simulink model "aa_IOT"  (R2024b)
settings: Solver=VariableStepAuto  StartTime=0.0  StopTime=0.20  RelTol=1e-3
undefined symbols (not defined in the file): Acid, Ion, Lead, Lithium, sigbuilder_block
libraries: spsBreakerLib x120, spsBatteryLib x72, spsSeriesRLCBranchLib x47, spsVoltageMeasurementLib x33, spsIdealSwitchLib x19, spsDiodeLib x10, spsCurrentMeasurementLib x8, spsThyristorLib x6, sldrtlib x4, spsACVoltageSourceLib x3, spsIGBTLib x2, spsPVArrayLib x1
(part 6 of 7)

== matlab function aa_IOT/Subsystem11/Swapping battery controller/MATLAB Function12 ==
  settings: updateMethod=DISCRETE
  data: SOC input; LoadOn output; ChargingOn output
function [LoadOn, ChargingOn] = chargeDischargeNode(SOC)
    % This function determines the charging and discharging states
    % based on the state of charge (SOC) of the battery.
    % Inputs:
    %   SOC - Current state of charge (0 to 100)
    % Outputs:
    %   LoadOn - Indicator if the load is on (1) or off (0)
    %   ChargingOn - Indicator if charging is active (1) or not (0)

    % Initialize persistent variables to retain state across function calls
    persistent LoadOnPersistent;
    persistent ChargingOnPersistent;

    if isempty(LoadOnPersistent)  % Initialize on first call
        LoadOnPersistent = 1;     % Load is initially on
        ChargingOnPersistent = 0;  % Charging is initially off
    end

    % Logic for charging and discharging based on SOC levels
    if SOC > 80
        LoadOnPersistent = 1;      % Turn load on if SOC is above 80%
        ChargingOnPersistent = 0;   % Turn charging off
    elseif SOC < 40
        LoadOnPersistent = 0;      % Turn load off if SOC is below 40%
        ChargingOnPersistent = 1;   % Start charging
    end

    % Assign output values from persistent variables
    LoadOn = LoadOnPersistent;
    ChargingOn = ChargingOnPersistent;
end

== matlab function aa_IOT/Subsystem11/Swapping battery controller/MATLAB Function13 ==
  settings: updateMethod=DISCRETE
  data: SOC input; LoadOn output; ChargingOn output
function [LoadOn, ChargingOn] = chargeDischargeNode(SOC)
    % This function determines the charging and discharging states
    % based on the state of charge (SOC) of the battery.
    % Inputs:
    %   SOC - Current state of charge (0 to 100)
    % Outputs:
    %   LoadOn - Indicator if the load is on (1) or off (0)
    %   ChargingOn - Indicator if charging is active (1) or not (0)

    % Initialize persistent variables to retain state across function calls
    persistent LoadOnPersistent;
    persistent ChargingOnPersistent;

    if isempty(LoadOnPersistent)  % Initialize on first call
        LoadOnPersistent = 1;     % Load is initially on
        ChargingOnPersistent = 0;  % Charging is initially off
    end

    % Logic for charging and discharging based on SOC levels
    if SOC > 80
        LoadOnPersistent = 1;      % Turn load on if SOC is above 80%
        ChargingOnPersistent = 0;   % Turn charging off
    elseif SOC < 40
        LoadOnPersistent = 0;      % Turn load off if SOC is below 40%
        ChargingOnPersistent = 1;   % Start charging
    end

    % Assign output values from persistent variables
    LoadOn = LoadOnPersistent;
    ChargingOn = ChargingOnPersistent;
end

== matlab function aa_IOT/Subsystem11/Swapping battery controller/MATLAB Function14 ==
  settings: updateMethod=DISCRETE
  data: SOC input; LoadOn output; ChargingOn output
function [LoadOn, ChargingOn] = chargeDischargeNode(SOC)
    % This function determines the charging and discharging states
    % based on the state of charge (SOC) of the battery.
    % Inputs:
    %   SOC - Current state of charge (0 to 100)
    % Outputs:
    %   LoadOn - Indicator if the load is on (1) or off (0)
    %   ChargingOn - Indicator if charging is active (1) or not (0)

    % Initialize persistent variables to retain state across function calls
    persistent LoadOnPersistent;
    persistent ChargingOnPersistent;

    if isempty(LoadOnPersistent)  % Initialize on first call
        LoadOnPersistent = 1;     % Load is initially on
        ChargingOnPersistent = 0;  % Charging is initially off
    end

    % Logic for charging and discharging based on SOC levels
    if SOC > 80
        LoadOnPersistent = 1;      % Turn load on if SOC is above 80%
        ChargingOnPersistent = 0;   % Turn charging off
    elseif SOC < 40
        LoadOnPersistent = 0;      % Turn load off if SOC is below 40%
        ChargingOnPersistent = 1;   % Start charging
    end

    % Assign output values from persistent variables
    LoadOn = LoadOnPersistent;
    ChargingOn = ChargingOnPersistent;
end

== matlab function aa_IOT/Subsystem11/Swapping battery controller/MATLAB Function15 ==
  settings: updateMethod=DISCRETE
  data: SOC input; LoadOn output; ChargingOn output
function [LoadOn, ChargingOn] = chargeDischargeNode(SOC)
    % This function determines the charging and discharging states
    % based on the state of charge (SOC) of the battery.
    % Inputs:
    %   SOC - Current state of charge (0 to 100)
    % Outputs:
    %   LoadOn - Indicator if the load is on (1) or off (0)
    %   ChargingOn - Indicator if charging is active (1) or not (0)

    % Initialize persistent variables to retain state across function calls
    persistent LoadOnPersistent;
    persistent ChargingOnPersistent;

    if isempty(LoadOnPersistent)  % Initialize on first call
        LoadOnPersistent = 1;     % Load is initially on
        ChargingOnPersistent = 0;  % Charging is initially off
    end

    % Logic for charging and discharging based on SOC levels
    if SOC > 80
        LoadOnPersistent = 1;      % Turn load on if SOC is above 80%
        ChargingOnPersistent = 0;   % Turn charging off
    elseif SOC < 40
        LoadOnPersistent = 0;      % Turn load off if SOC is below 40%
        ChargingOnPersistent = 1;   % Start charging
    end

    % Assign output values from persistent variables
    LoadOn = LoadOnPersistent;
    ChargingOn = ChargingOnPersistent;
end

== matlab function aa_IOT/Subsystem11/Swapping battery controller/MATLAB Function16 ==
  settings: updateMethod=DISCRETE
  data: SOC input; LoadOn output; ChargingOn output
function [LoadOn, ChargingOn] = chargeDischargeNode(SOC)
    % This function determines the charging and discharging states
    % based on the state of charge (SOC) of the battery.
    % Inputs:
    %   SOC - Current state of charge (0 to 100)
    % Outputs:
    %   LoadOn - Indicator if the load is on (1) or off (0)
    %   ChargingOn - Indicator if charging is active (1) or not (0)

    % Initialize persistent variables to retain state across function calls
    persistent LoadOnPersistent;
    persistent ChargingOnPersistent;

    if isempty(LoadOnPersistent)  % Initialize on first call
        LoadOnPersistent = 1;     % Load is initially on
        ChargingOnPersistent = 0;  % Charging is initially off
    end

    % Logic for charging and discharging based on SOC levels
    if SOC > 80
        LoadOnPersistent = 1;      % Turn load on if SOC is above 80%
        ChargingOnPersistent = 0;   % Turn charging off
    elseif SOC < 40
        LoadOnPersistent = 0;      % Turn load off if SOC is below 40%
        ChargingOnPersistent = 1;   % Start charging
    end

    % Assign output values from persistent variables
    LoadOn = LoadOnPersistent;
    ChargingOn = ChargingOnPersistent;
end

== matlab function aa_IOT/Subsystem11/Swapping battery controller/MATLAB Function17 ==
  settings: updateMethod=DISCRETE
  data: SOC input; LoadOn output; ChargingOn output
function [LoadOn, ChargingOn] = chargeDischargeNode(SOC)
    % This function determines the charging and discharging states
    % based on the state of charge (SOC) of the battery.
    % Inputs:
    %   SOC - Current state of charge (0 to 100)
    % Outputs:
    %   LoadOn - Indicator if the load is on (1) or off (0)
    %   ChargingOn - Indicator if charging is active (1) or not (0)

    % Initialize persistent variables to retain state across function calls
    persistent LoadOnPersistent;
    persistent ChargingOnPersistent;

    if isempty(LoadOnPersistent)  % Initialize on first call
        LoadOnPersistent = 1;     % Load is initially on
        ChargingOnPersistent = 0;  % Charging is initially off
    end

    % Logic for charging and discharging based on SOC levels
    if SOC > 80
        LoadOnPersistent = 1;      % Turn load on if SOC is above 80%
        ChargingOnPersistent = 0;   % Turn charging off
    elseif SOC < 40
        LoadOnPersistent = 0;      % Turn load off if SOC is below 40%
        ChargingOnPersistent = 1;   % Start charging
    end

    % Assign output values from persistent variables
    LoadOn = LoadOnPersistent;
    ChargingOn = ChargingOnPersistent;
end

== matlab function aa_IOT/Subsystem11/Swapping battery controller/MATLAB Function18 ==
  settings: updateMethod=DISCRETE
  data: SOC input; LoadOn output; ChargingOn output
function [LoadOn, ChargingOn] = chargeDischargeNode(SOC)
    % This function determines the charging and discharging states
    % based on the state of charge (SOC) of the battery.
    % Inputs:
    %   SOC - Current state of charge (0 to 100)
    % Outputs:
    %   LoadOn - Indicator if the load is on (1) or off (0)
    %   ChargingOn - Indicator if charging is active (1) or not (0)

    % Initialize persistent variables to retain state across function calls
    persistent LoadOnPersistent;
    persistent ChargingOnPersistent;

    if isempty(LoadOnPersistent)  % Initialize on first call
        LoadOnPersistent = 1;     % Load is initially on
        ChargingOnPersistent = 0;  % Charging is initially off
    end

    % Logic for charging and discharging based on SOC levels
    if SOC > 80
        LoadOnPersistent = 1;      % Turn load on if SOC is above 80%
        ChargingOnPersistent = 0;   % Turn charging off
    elseif SOC < 40
        LoadOnPersistent = 0;      % Turn load off if SOC is below 40%
        ChargingOnPersistent = 1;   % Start charging
    end

    % Assign output values from persistent variables
    LoadOn = LoadOnPersistent;
    ChargingOn = ChargingOnPersistent;
end

== matlab function aa_IOT/Subsystem11/Swapping battery controller/MATLAB Function19 ==
  settings: updateMethod=DISCRETE
  data: SOC input; LoadOn output; ChargingOn output
function [LoadOn, ChargingOn] = chargeDischargeNode(SOC)
    % This function determines the charging and discharging states
    % based on the state of charge (SOC) of the battery.
    % Inputs:
    %   SOC - Current state of charge (0 to 100)
    % Outputs:
    %   LoadOn - Indicator if the load is on (1) or off (0)
    %   ChargingOn - Indicator if charging is active (1) or not (0)

    % Initialize persistent variables to retain state across function calls
    persistent LoadOnPersistent;
    persistent ChargingOnPersistent;

    if isempty(LoadOnPersistent)  % Initialize on first call
        LoadOnPersistent = 1;     % Load is initially on
        ChargingOnPersistent = 0;  % Charging is initially off
    end

    % Logic for charging and discharging based on SOC levels
    if SOC > 80
        LoadOnPersistent = 1;      % Turn load on if SOC is above 80%
        ChargingOnPersistent = 0;   % Turn charging off
    elseif SOC < 40
        LoadOnPersistent = 0;      % Turn load off if SOC is below 40%
        ChargingOnPersistent = 1;   % Start charging
    end

    % Assign output values from persistent variables
    LoadOn = LoadOnPersistent;
    ChargingOn = ChargingOnPersistent;
end

== matlab function aa_IOT/Subsystem11/Swapping battery controller/MATLAB Function20 ==
  settings: updateMethod=DISCRETE
  data: SOC input; LoadOn output; ChargingOn output
function [LoadOn, ChargingOn] = chargeDischargeNode(SOC)
    % This function determines the charging and discharging states
    % based on the state of charge (SOC) of the battery.
    % Inputs:
    %   SOC - Current state of charge (0 to 100)
    % Outputs:
    %   LoadOn - Indicator if the load is on (1) or off (0)
    %   ChargingOn - Indicator if charging is active (1) or not (0)

    % Initialize persistent variables to retain state across function calls
    persistent LoadOnPersistent;
    persistent ChargingOnPersistent;

    if isempty(LoadOnPersistent)  % Initialize on first call
        LoadOnPersistent = 1;     % Load is initially on
        ChargingOnPersistent = 0;  % Charging is initially off
    end

    % Logic for charging and discharging based on SOC levels
    if SOC > 80
        LoadOnPersistent = 1;      % Turn load on if SOC is above 80%
        ChargingOnPersistent = 0;   % Turn charging off
    elseif SOC < 40
        LoadOnPersistent = 0;      % Turn load off if SOC is below 40%
        ChargingOnPersistent = 1;   % Start charging
    end

    % Assign output values from persistent variables
    LoadOn = LoadOnPersistent;
    ChargingOn = ChargingOnPersistent;
end

== matlab function aa_IOT/Subsystem11/Swapping battery controller/MATLAB Function21 ==
  settings: updateMethod=DISCRETE
  data: SOC input; LoadOn output; ChargingOn output
function [LoadOn, ChargingOn] = chargeDischargeNode(SOC)
    % This function determines the charging and discharging states
    % based on the state of charge (SOC) of the battery.
    % Inputs:
    %   SOC - Current state of charge (0 to 100)
    % Outputs:
    %   LoadOn - Indicator if the load is on (1) or off (0)
    %   ChargingOn - Indicator if charging is active (1) or not (0)

    % Initialize persistent variables to retain state across function calls
    persistent LoadOnPersistent;
    persistent ChargingOnPersistent;

    if isempty(LoadOnPersistent)  % Initialize on first call
        LoadOnPersistent = 1;     % Load is initially on
        ChargingOnPersistent = 0;  % Charging is initially off
    end

    % Logic for charging and discharging based on SOC levels
    if SOC > 80
        LoadOnPersistent = 1;      % Turn load on if SOC is above 80%
        ChargingOnPersistent = 0;   % Turn charging off
    elseif SOC < 40
        LoadOnPersistent = 0;      % Turn load off if SOC is below 40%
        ChargingOnPersistent = 1;   % Start charging
    end

    % Assign output values from persistent variables
    LoadOn = LoadOnPersistent;
    ChargingOn = ChargingOnPersistent;
end

== matlab function aa_IOT/Subsystem11/Swapping battery controller/MATLAB Function22 ==
  settings: updateMethod=DISCRETE
  data: SOC input; LoadOn output; ChargingOn output
function [LoadOn, ChargingOn] = chargeDischargeNode(SOC)
    % This function determines the charging and discharging states
    % based on the state of charge (SOC) of the battery.
    % Inputs:
    %   SOC - Current state of charge (0 to 100)
    % Outputs:
    %   LoadOn - Indicator if the load is on (1) or off (0)
    %   ChargingOn - Indicator if charging is active (1) or not (0)

    % Initialize persistent variables to retain state across function calls
    persistent LoadOnPersistent;
    persistent ChargingOnPersistent;

    if isempty(LoadOnPersistent)  % Initialize on first call
        LoadOnPersistent = 1;     % Load is initially on
        ChargingOnPersistent = 0;  % Charging is initially off
    end

    % Logic for charging and discharging based on SOC levels
    if SOC > 80
        LoadOnPersistent = 1;      % Turn load on if SOC is above 80%
        ChargingOnPersistent = 0;   % Turn charging off
    elseif SOC < 40
        LoadOnPersistent = 0;      % Turn load off if SOC is below 40%
        ChargingOnPersistent = 1;   % Start charging
    end

    % Assign output values from persistent variables
    LoadOn = LoadOnPersistent;
    ChargingOn = ChargingOnPersistent;
end

== matlab function aa_IOT/Subsystem11/Subsystem5/MATLAB Function ==
  data: SOC input; output output; Voltage input; Current input
function output = checkBatteryStatus(SOC, Voltage, Current)
    % Check if the inputs are valid
    if SOC <= 0 || Voltage <= 0 || Current <= 0
        output = 0; % Return 0 if any input is less than or equal to 0
        return;
    end
    
    % Define threshold values
    SOC_threshold = 80; % in percentage
    Voltage_threshold = 10; % in volts
    Current_threshold = 13; % in amperes

    % Check conditions and return output
    if SOC > SOC_threshold && Voltage > Voltage_threshold && Current > Current_threshold
        output = 0; % Return 0 if all conditions are met
    else
        output = 1; % Return 1 otherwise
    end
end

== matlab function aa_IOT/Subsystem11/Swapping battery controller/MATLAB Function23 ==
  settings: updateMethod=DISCRETE
  data: SOC input; LoadOn output; ChargingOn output
function [LoadOn, ChargingOn] = chargeDischargeNode(SOC)
    % This function determines the charging and discharging states
    % based on the state of charge (SOC) of the battery.
    % Inputs:
    %   SOC - Current state of charge (0 to 100)
    % Outputs:
    %   LoadOn - Indicator if the load is on (1) or off (0)
    %   ChargingOn - Indicator if charging is active (1) or not (0)

    % Initialize persistent variables to retain state across function calls
    persistent LoadOnPersistent;
    persistent ChargingOnPersistent;

    if isempty(LoadOnPersistent)  % Initialize on first call
        LoadOnPersistent = 1;     % Load is initially on
        ChargingOnPersistent = 0;  % Charging is initially off
    end

    % Logic for charging and discharging based on SOC levels
    if SOC > 80
        LoadOnPersistent = 1;      % Turn load on if SOC is above 80%
        ChargingOnPersistent = 0;   % Turn charging off
    elseif SOC < 40
        LoadOnPersistent = 0;      % Turn load off if SOC is below 40%
        ChargingOnPersistent = 1;   % Start charging
    end

    % Assign output values from persistent variables
    LoadOn = LoadOnPersistent;
    ChargingOn = ChargingOnPersistent;
end

== matlab function aa_IOT/Subsystem11/Swapping battery controller/MATLAB Function24 ==
  settings: updateMethod=DISCRETE
  data: SOC input; LoadOn output; ChargingOn output
function [LoadOn, ChargingOn] = chargeDischargeNode(SOC)
    % This function determines the charging and discharging states
    % based on the state of charge (SOC) of the battery.
    % Inputs:
    %   SOC - Current state of charge (0 to 100)
    % Outputs:
    %   LoadOn - Indicator if the load is on (1) or off (0)
    %   ChargingOn - Indicator if charging is active (1) or not (0)

    % Initialize persistent variables to retain state across function calls
    persistent LoadOnPersistent;
    persistent ChargingOnPersistent;

    if isempty(LoadOnPersistent)  % Initialize on first call
        LoadOnPersistent = 1;     % Load is initially on
        ChargingOnPersistent = 0;  % Charging is initially off
    end

    % Logic for charging and discharging based on SOC levels
    if SOC > 80
        LoadOnPersistent = 1;      % Turn load on if SOC is above 80%
        ChargingOnPersistent = 0;   % Turn charging off
    elseif SOC < 40
        LoadOnPersistent = 0;      % Turn load off if SOC is below 40%
        ChargingOnPersistent = 1;   % Start charging
    end

    % Assign output values from persistent variables
    LoadOn = LoadOnPersistent;
    ChargingOn = ChargingOnPersistent;
end

== matlab function aa_IOT/Subsystem11/Swapping battery controller/MATLAB Function25 ==
  settings: updateMethod=DISCRETE
  data: SOC input; LoadOn output; ChargingOn output
function [LoadOn, ChargingOn] = chargeDischargeNode(SOC)
    % This function determines the charging and discharging states
    % based on the state of charge (SOC) of the battery.
    % Inputs:
    %   SOC - Current state of charge (0 to 100)
    % Outputs:
    %   LoadOn - Indicator if the load is on (1) or off (0)
    %   ChargingOn - Indicator if charging is active (1) or not (0)

    % Initialize persistent variables to retain state across function calls
    persistent LoadOnPersistent;
    persistent ChargingOnPersistent;

    if isempty(LoadOnPersistent)  % Initialize on first call
        LoadOnPersistent = 1;     % Load is initially on
        ChargingOnPersistent = 0;  % Charging is initially off
    end

    % Logic for charging and discharging based on SOC levels
    if SOC > 80
        LoadOnPersistent = 1;      % Turn load on if SOC is above 80%
        ChargingOnPersistent = 0;   % Turn charging off
    elseif SOC < 40
        LoadOnPersistent = 0;      % Turn load off if SOC is below 40%
        ChargingOnPersistent = 1;   % Start charging
    end

    % Assign output values from persistent variables
    LoadOn = LoadOnPersistent;
    ChargingOn = ChargingOnPersistent;
end

== matlab function aa_IOT/Subsystem11/Swapping battery controller/MATLAB Function26 ==
  settings: updateMethod=DISCRETE
  data: SOC input; LoadOn output; ChargingOn output
function [LoadOn, ChargingOn] = chargeDischargeNode(SOC)
    % This function determines the charging and discharging states
    % based on the state of charge (SOC) of the battery.
    % Inputs:
    %   SOC - Current state of charge (0 to 100)
    % Outputs:
    %   LoadOn - Indicator if the load is on (1) or off (0)
    %   ChargingOn - Indicator if charging is active (1) or not (0)

    % Initialize persistent variables to retain state across function calls
    persistent LoadOnPersistent;
    persistent ChargingOnPersistent;

    if isempty(LoadOnPersistent)  % Initialize on first call
        LoadOnPersistent = 1;     % Load is initially on
        ChargingOnPersistent = 0;  % Charging is initially off
    end

    % Logic for charging and discharging based on SOC levels
    if SOC > 80
        LoadOnPersistent = 1;      % Turn load on if SOC is above 80%
        ChargingOnPersistent = 0;   % Turn charging off
    elseif SOC < 40
        LoadOnPersistent = 0;      % Turn load off if SOC is below 40%
        ChargingOnPersistent = 1;   % Start charging
    end

    % Assign output values from persistent variables
    LoadOn = LoadOnPersistent;
    ChargingOn = ChargingOnPersistent;
end

== matlab function aa_IOT/Subsystem11/Swapping battery controller/MATLAB Function27 ==
  settings: updateMethod=DISCRETE
  data: SOC input; LoadOn output; ChargingOn output
function [LoadOn, ChargingOn] = chargeDischargeNode(SOC)
    % This function determines the charging and discharging states
    % based on the state of charge (SOC) of the battery.
    % Inputs:
    %   SOC - Current state of charge (0 to 100)
    % Outputs:
    %   LoadOn - Indicator if the load is on (1) or off (0)
    %   ChargingOn - Indicator if charging is active (1) or not (0)

    % Initialize persistent variables to retain state across function calls
    persistent LoadOnPersistent;
    persistent ChargingOnPersistent;

    if isempty(LoadOnPersistent)  % Initialize on first call
        LoadOnPersistent = 1;     % Load is initially on
        ChargingOnPersistent = 0;  % Charging is initially off
    end

    % Logic for charging and discharging based on SOC levels
    if SOC > 80
        LoadOnPersistent = 1;      % Turn load on if SOC is above 80%
        ChargingOnPersistent = 0;   % Turn charging off
    elseif SOC < 40
        LoadOnPersistent = 0;      % Turn load off if SOC is below 40%
        ChargingOnPersistent = 1;   % Start charging
    end

    % Assign output values from persistent variables
    LoadOn = LoadOnPersistent;
    ChargingOn = ChargingOnPersistent;
end

== matlab function aa_IOT/Subsystem11/Swapping battery controller/MATLAB Function28 ==
  settings: updateMethod=DISCRETE
  data: SOC input; LoadOn output; ChargingOn output
function [LoadOn, ChargingOn] = chargeDischargeNode(SOC)
    % This function determines the charging and discharging states
    % based on the state of charge (SOC) of the battery.
    % Inputs:
    %   SOC - Current state of charge (0 to 100)
    % Outputs:
    %   LoadOn - Indicator if the load is on (1) or off (0)
    %   ChargingOn - Indicator if charging is active (1) or not (0)

    % Initialize persistent variables to retain state across function calls
    persistent LoadOnPersistent;
    persistent ChargingOnPersistent;

    if isempty(LoadOnPersistent)  % Initialize on first call
        LoadOnPersistent = 1;     % Load is initially on
        ChargingOnPersistent = 0;  % Charging is initially off
    end

    % Logic for charging and discharging based on SOC levels
    if SOC > 80
        LoadOnPersistent = 1;      % Turn load on if SOC is above 80%
        ChargingOnPersistent = 0;   % Turn charging off
    elseif SOC < 40
        LoadOnPersistent = 0;      % Turn load off if SOC is below 40%
        ChargingOnPersistent = 1;   % Start charging
    end

    % Assign output values from persistent variables
    LoadOn = LoadOnPersistent;
    ChargingOn = ChargingOnPersistent;
end

== matlab function aa_IOT/Subsystem11/Swapping battery controller/MATLAB Function29 ==
  settings: updateMethod=DISCRETE
  data: SOC input; LoadOn output; ChargingOn output
function [LoadOn, ChargingOn] = chargeDischargeNode(SOC)
    % This function determines the charging and discharging states
    % based on the state of charge (SOC) of the battery.
    % Inputs:
    %   SOC - Current state of charge (0 to 100)
    % Outputs:
    %   LoadOn - Indicator if the load is on (1) or off (0)
    %   ChargingOn - Indicator if charging is active (1) or not (0)

    % Initialize persistent variables to retain state across function calls
    persistent LoadOnPersistent;
    persistent ChargingOnPersistent;

    if isempty(LoadOnPersistent)  % Initialize on first call
        LoadOnPersistent = 1;     % Load is initially on
        ChargingOnPersistent = 0;  % Charging is initially off
    end

    % Logic for charging and discharging based on SOC levels
    if SOC > 80
        LoadOnPersistent = 1;      % Turn load on if SOC is above 80%
        ChargingOnPersistent = 0;   % Turn charging off
    elseif SOC < 40
        LoadOnPersistent = 0;      % Turn load off if SOC is below 40%
        ChargingOnPersistent = 1;   % Start charging
    end

    % Assign output values from persistent variables
    LoadOn = LoadOnPersistent;
    ChargingOn = ChargingOnPersistent;
end

== matlab function aa_IOT/Subsystem11/Subsystem3/MATLAB Function ==
  data: SOC input; output output; Voltage input; Current input
function output = checkBatteryStatus(SOC, Voltage, Current)
    % Check if the inputs are valid
    if SOC <= 0 || Voltage <= 0 || Current <= 0
        output = 0; % Return 0 if any input is less than or equal to 0
        return;
    end
    
    % Define threshold values
    SOC_threshold = 80; % in percentage
    Voltage_threshold = 10; % in volts
    Current_threshold = 13; % in amperes

    % Check conditions and return output
    if SOC > SOC_threshold && Voltage > Voltage_threshold && Current > Current_threshold
        output = 0; % Return 0 if all conditions are met
    else
        output = 1; % Return 1 otherwise
    end
end

== matlab function aa_IOT/Subsystem11/Subsystem2/MATLAB Function ==
  data: SOC input; output output; Voltage input; Current input
function output = checkBatteryStatus(SOC, Voltage, Current)
    % Check if the inputs are valid
    if SOC <= 0 || Voltage <= 0 || Current <= 0
        output = 0; % Return 0 if any input is less than or equal to 0
        return;
    end
    
    % Define threshold values
    SOC_threshold = 80; % in percentage
    Voltage_threshold = 10; % in volts
    Current_threshold = 13; % in amperes

    % Check conditions and return output
    if SOC > SOC_threshold && Voltage > Voltage_threshold && Current > Current_threshold
        output = 0; % Return 0 if all conditions are met
    else
        output = 1; % Return 1 otherwise
    end
end

== matlab function aa_IOT/Subsystem11/Subsystem20/MATLAB Function ==
  data: SOC input; output output; Voltage input; Current input
function output = checkBatteryStatus(SOC, Voltage, Current)
    % Check if the inputs are valid
    if SOC <= 0 || Voltage <= 0 || Current <= 0
        output = 0; % Return 0 if any input is less than or equal to 0
        return;
    end
    
    % Define threshold values
    SOC_threshold = 80; % in percentage
    Voltage_threshold = 10; % in volts
    Current_threshold = 13; % in amperes

    % Check conditions and return output
    if SOC > SOC_threshold && Voltage > Voltage_threshold && Current > Current_threshold
        output = 0; % Return 0 if all conditions are met
    else
        output = 1; % Return 1 otherwise
    end
end

== matlab function aa_IOT/Subsystem11/Subsystem19/MATLAB Function ==
  data: SOC input; output output; Voltage input; Current input
function output = checkBatteryStatus(SOC, Voltage, Current)
    % Check if the inputs are valid
    if SOC <= 0 || Voltage <= 0 || Current <= 0
        output = 0; % Return 0 if any input is less than or equal to 0
        return;
    end
    
    % Define threshold values
    SOC_threshold = 80; % in percentage
    Voltage_threshold = 10; % in volts
    Current_threshold = 13; % in amperes

    % Check conditions and return output
    if SOC > SOC_threshold && Voltage > Voltage_threshold && Current > Current_threshold
        output = 0; % Return 0 if all conditions are met
    else
        output = 1; % Return 1 otherwise
    end
end

== matlab function aa_IOT/Solar/MPPT/Embedded MATLAB Function1 ==
  settings: updateMethod=DISCRETE
  data: V input; I input; T input; D output
function D   = PO(V,I,T)
persistent P2  P1  dP d dd n;
if isempty(V)
    V=370;
end
if isempty(I)
    I=0;
end
if isempty(P2)
    P2=0;
end
if isempty(P1)
    P1=0;
end
if isempty(dP)
    dP=0;
end
if isempty(d)
    d=1;
end
if isempty(dd)
    dd=0;
end
if isempty(n)
    n=1;
end
%%%%%%%%%%%%%%%%%%%%%
    if  (T > n*0.02)   %chu ki lay mau 0.02s
    n = n + 1;
    P1=P2;
    P2=V*I;
    dP=P2-P1;
    if (dd==0)
        if dP>1
            dd=0.01;
            d=d+dd;
        else
            if dP<-1
                dd=-0.01;
                d=d+dd;
            else
                dd=0;
            end
        end
    else
        if ((dP<1)&&(dP>-1))
        dd=0;
        d=d+dd;
        else
            if ((dP/dd)>0)
                dd=0.01;
                d=d+dd;
            else
                dd=-0.01;
                d=d+dd;
            end
        end
    end    
    end
D=d/(d+1);
if D<0.4
    D=0.4;
    d=D/(1-D);
else
    if D>0.9
        D=0.9;
        d=D/(1-D);
    else
    end
end
end

== matlab function aa_IOT/Subsystem11/Subsystem15/MATLAB Function ==
  data: SOC input; output output; Voltage input; Current input
function output = checkBatteryStatus(SOC, Voltage, Current)
    % Check if the inputs are valid
    if SOC <= 0 || Voltage <= 0 || Current <= 0
        output = 0; % Return 0 if any input is less than or equal to 0
        return;
    end
    
    % Define threshold values
    SOC_threshold = 80; % in percentage
    Voltage_threshold = 10; % in volts
    Current_threshold = 13; % in amperes

    % Check conditions and return output
    if SOC > SOC_threshold && Voltage > Voltage_threshold && Current > Current_threshold
        output = 0; % Return 0 if all conditions are met
    else
        output = 1; % Return 1 otherwise
    end
end

== matlab function aa_IOT/Subsystem11/Subsystem13/MATLAB Function ==
  data: SOC input; output output; Voltage input; Current input
function output = checkBatteryStatus(SOC, Voltage, Current)
    % Check if the inputs are valid
    if SOC <= 0 || Voltage <= 0 || Current <= 0
        output = 0; % Return 0 if any input is less than or equal to 0
        return;
    end
    
    % Define threshold values
    SOC_threshold = 80; % in percentage
    Voltage_threshold = 10; % in volts
    Current_threshold = 13; % in amperes

    % Check conditions and return output
    if SOC > SOC_threshold && Voltage > Voltage_threshold && Current > Current_threshold
        output = 0; % Return 0 if all conditions are met
    else
        output = 1; % Return 1 otherwise
    end
end

== matlab function aa_IOT/Subsystem11/Subsystem10/MATLAB Function ==
  data: SOC input; output output; Voltage input; Current input
function output = checkBatteryStatus(SOC, Voltage, Current)
    % Check if the inputs are valid
    if SOC <= 0 || Voltage <= 0 || Current <= 0
        output = 0; % Return 0 if any input is less than or equal to 0
        return;
    end
    
    % Define threshold values
    SOC_threshold = 80; % in percentage
    Voltage_threshold = 10; % in volts
    Current_threshold = 13; % in amperes

    % Check conditions and return output
    if SOC > SOC_threshold && Voltage > Voltage_threshold && Current > Current_threshold
        output = 0; % Return 0 if all conditions are met
    else
        output = 1; % Return 1 otherwise
    end
end

== matlab function aa_IOT/Subsystem11/Subsystem11/MATLAB Function ==
  data: SOC input; output output; Voltage input; Current input
function output = checkBatteryStatus(SOC, Voltage, Current)
    % Check if the inputs are valid
    if SOC <= 0 || Voltage <= 0 || Current <= 0
        output = 0; % Return 0 if any input is less than or equal to 0
        return;
    end
    
    % Define threshold values
    SOC_threshold = 80; % in percentage
    Voltage_threshold = 10; % in volts
    Current_threshold = 13; % in amperes

    % Check conditions and return output
    if SOC > SOC_threshold && Voltage > Voltage_threshold && Current > Current_threshold
        output = 0; % Return 0 if all conditions are met
    else
        output = 1; % Return 1 otherwise
    end
end

== matlab function aa_IOT/Subsystem11/Subsystem9/MATLAB Function ==
  data: SOC input; output output; Voltage input; Current input
function output = checkBatteryStatus(SOC, Voltage, Current)
    % Check if the inputs are valid
    if SOC <= 0 || Voltage <= 0 || Current <= 0
        output = 0; % Return 0 if any input is less than or equal to 0
        return;
    end
    
    % Define threshold values
    SOC_threshold = 80; % in percentage
    Voltage_threshold = 10; % in volts
    Current_threshold = 13; % in amperes

    % Check conditions and return output
    if SOC > SOC_threshold && Voltage > Voltage_threshold && Current > Current_threshold
        output = 0; % Return 0 if all conditions are met
    else
        output = 1; % Return 1 otherwise
    end
end

== matlab function aa_IOT/Subsystem11/Subsystem29/MATLAB Function ==
  data: SOC input; output output; Voltage input; Current input
function output = checkBatteryStatus(SOC, Voltage, Current)
    % Check if the inputs are valid
    if SOC <= 0 || Voltage <= 0 || Current <= 0
        output = 0; % Return 0 if any input is less than or equal to 0
        return;
    end
    
    % Define threshold values
    SOC_threshold = 80; % in percentage
    Voltage_threshold = 10; % in volts
    Current_threshold = 13; % in amperes

    % Check conditions and return output
    if SOC > SOC_threshold && Voltage > Voltage_threshold && Current > Current_threshold
        output = 0; % Return 0 if all conditions are met
    else
        output = 1; % Return 1 otherwise
    end
end

== matlab function aa_IOT/Subsystem11/Subsystem27/MATLAB Function ==
  data: SOC input; output output; Voltage input; Current input
function output = checkBatteryStatus(SOC, Voltage, Current)
    % Check if the inputs are valid
    if SOC <= 0 || Voltage <= 0 || Current <= 0
        output = 0; % Return 0 if any input is less than or equal to 0
        return;
    end
    
    % Define threshold values
    SOC_threshold = 80; % in percentage
    Voltage_threshold = 10; % in volts
    Current_threshold = 13; % in amperes

    % Check conditions and return output
    if SOC > SOC_threshold && Voltage > Voltage_threshold && Current > Current_threshold
        output = 0; % Return 0 if all conditions are met
    else
        output = 1; % Return 1 otherwise
    end
end

== matlab function aa_IOT/Subsystem11/Subsystem24/MATLAB Function ==
  data: SOC input; output output; Voltage input; Current input
function output = checkBatteryStatus(SOC, Voltage, Current)
    % Check if the inputs are valid
    if SOC <= 0 || Voltage <= 0 || Current <= 0
        output = 0; % Return 0 if any input is less than or equal to 0
        return;
    end
    
    % Define threshold values
    SOC_threshold = 80; % in percentage
    Voltage_threshold = 10; % in volts
    Current_threshold = 13; % in amperes

    % Check conditions and return output
    if SOC > SOC_threshold && Voltage > Voltage_threshold && Current > Current_threshold
        output = 0; % Return 0 if all conditions are met
    else
        output = 1; % Return 1 otherwise
    end
end

== matlab function aa_IOT/Subsystem11/Subsystem25/MATLAB Function ==
  data: SOC input; output output; Voltage input; Current input
function output = checkBatteryStatus(SOC, Voltage, Current)
    % Check if the inputs are valid
    if SOC <= 0 || Voltage <= 0 || Current <= 0
        output = 0; % Return 0 if any input is less than or equal to 0
        return;
    end
    
    % Define threshold values
    SOC_threshold = 80; % in percentage
    Voltage_threshold = 10; % in volts
    Current_threshold = 13; % in amperes

    % Check conditions and return output
    if SOC > SOC_threshold && Voltage > Voltage_threshold && Current > Current_threshold
        output = 0; % Return 0 if all conditions are met
    else
        output = 1; % Return 1 otherwise
    end
end

== matlab function aa_IOT/Subsystem11/Subsystem23/MATLAB Function ==
  data: SOC input; output output; Voltage input; Current input
function output = checkBatteryStatus(SOC, Voltage, Current)
    % Check if the inputs are valid
    if SOC <= 0 || Voltage <= 0 || Current <= 0
        output = 0; % Return 0 if any input is less than or equal to 0
        return;
    end
    
    % Define threshold values
    SOC_threshold = 80; % in percentage
    Voltage_threshold = 10; % in volts
    Current_threshold = 13; % in amperes

    % Check conditions and return output
    if SOC > SOC_threshold && Voltage > Voltage_threshold && Current > Current_threshold
        output = 0; % Return 0 if all conditions are met
    else
        output = 1; % Return 1 otherwise
    end
end

== matlab function aa_IOT/Subsystem11/Swapping battery controller/MATLAB Function ==
  settings: updateMethod=DISCRETE
  data: SOC input; LoadOn output; ChargingOn output
function [LoadOn, ChargingOn] = chargeDischargeNode(SOC)
    % This function determines the charging and discharging states
    % based on the state of charge (SOC) of the battery.
    % Inputs:
    %   SOC - Current state of charge (0 to 100)
    % Outputs:
    %   LoadOn - Indicator if the load is on (1) or off (0)
    %   ChargingOn - Indicator if charging is active (1) or not (0)

    % Initialize persistent variables to retain state across function calls
    persistent LoadOnPersistent;
    persistent ChargingOnPersistent;

    if isempty(LoadOnPersistent)  % Initialize on first call
        LoadOnPersistent = 1;     % Load is initially on
        ChargingOnPersistent = 0;  % Charging is initially off
    end

    % Logic for charging and discharging based on SOC levels
    if SOC > 80
        LoadOnPersistent = 1;      % Turn load on if SOC is above 80%
        ChargingOnPersistent = 0;   % Turn charging off
    elseif SOC < 40
        LoadOnPersistent = 0;      % Turn load off if SOC is below 40%
        ChargingOnPersistent = 1;   % Start charging
    end

    % Assign output values from persistent variables
    LoadOn = LoadOnPersistent;
    ChargingOn = ChargingOnPersistent;
end

== matlab function aa_IOT/Subsystem3/MATLAB Function ==
  data: voltage input; voltageLevel output; current input; temperature input; currentLevel output; SOC output; SOH output; DOD output; ROH output; batteryLifeCycle output; insulationResistance output; residualCurrentMonitoring output; temperatureMonitoring output; chargingTime output
function [voltageLevel, currentLevel, SOC, SOH, DOD, ROH, batteryLifeCycle, insulationResistance, residualCurrentMonitoring, temperatureMonitoring, chargingTime] = BatteryParameterEstimation(voltage, current, temperature)
    % BatteryParameterEstimation calculates various battery parameters based on voltage, current, and temperature.
    %
    % Inputs:
    %   voltage - The voltage of the battery in volts
    %   current - The current flowing into the battery in amperes
    %   temperature - The temperature of the battery in degrees Celsius
    %
    % Outputs:
    %   voltageLevel - Monitored voltage level
    %   currentLevel - Monitored current level
    %   SOC - State of Charge as a percentage
    %   SOH - State of Health as a percentage
    %   DOD - Depth of Discharge as a percentage
    %   ROH - Remaining Operating Hours
    %   batteryLifeCycle - Estimated remaining battery life cycles
    %   insulationResistance - Insulation resistance in ohms (example constant)
    %   residualCurrentMonitoring - Boolean indicating overcurrent condition
    %   temperatureMonitoring - Monitored temperature value
    %   chargingTime - Estimated charging time in hours

    % Constants for calculations (these values are examples and may need to be adjusted)
    nominalVoltage = 12;        % Nominal voltage of the battery in volts
    maxCurrent = 100;           % Maximum current rating in amperes
    fullChargeCapacity = 100;   % Full charge capacity in Ah
    minVoltageCutoff = 10.5;    % Minimum voltage cutoff for the battery in volts
    maxCycles = 500;            % Estimated maximum cycles for the battery life

    %% 1. Voltage Levels
    voltageLevel = voltage;

    %% 2. Current Levels
    currentLevel = current;

    %% 3. State of Charge (SOC) Calculation
    SOC = (voltage - minVoltageCutoff) / (nominalVoltage - minVoltageCutoff) * 100;
    SOC = max(0, min(SOC, 100));  % Ensure SOC is between 0% and 100%

    %% 4. State of Health (SOH) Calculation (example based on voltage drop)
    SOH = (voltage / nominalVoltage) * 100;

    %% 5. Depth of Discharge (DOD) Calculation
    DOD = 100 - SOC;  % DOD is the complement of SOC

    %% 6. Remaining Operating Hours (ROH) Calculation
    ROH = (fullChargeCapacity - (current / fullChargeCapacity)) * fullChargeCapacity / current; 
    ROH = max(0, ROH);  % Ensure ROH is not negative

    %% 7. Battery Life Cycle Calculation
    batteryLifeCycle = maxCycles * (SOC / 100);  % Estimate remaining cycles based on SOC

    %% 8. Insulation Resistance Calculation (example constant)
    insulationResistance = 1000;  % Example value in ohms

    %% 9. Residual Current Monitoring Calculation (example condition)
    residualCurrentMonitoring = current > maxCurrent;  % True if overcurrent condition

    %% 10. Temperature Monitoring
    temperatureMonitoring = temperature;  % Directly use temperature input

    %% 11. Charging Time Calculation (example)
    chargingTime = (fullChargeCapacity - DOD * fullChargeCapacity / 100) / current; 
end

== matlab function aa_IOT/Subsystem2/MATLAB Function ==
  data: voltage input; voltageLevel output; current input; temperature input; currentLevel output; SOC output; SOH output; DOD output; ROH output; batteryLifeCycle output; insulationResistance output; residualCurrentMonitoring output; temperatureMonitoring output; chargingTime output
function [voltageLevel, currentLevel, SOC, SOH, DOD, ROH, batteryLifeCycle, insulationResistance, residualCurrentMonitoring, temperatureMonitoring, chargingTime] = BatteryParameterEstimation(voltage, current, temperature)
    % BatteryParameterEstimation calculates various battery parameters based on voltage, current, and temperature.
    %
    % Inputs:
    %   voltage - The voltage of the battery in volts
    %   current - The current flowing into the battery in amperes
    %   temperature - The temperature of the battery in degrees Celsius
    %
    % Outputs:
    %   voltageLevel - Monitored voltage level
    %   currentLevel - Monitored current level
    %   SOC - State of Charge as a percentage
    %   SOH - State of Health as a percentage
    %   DOD - Depth of Discharge as a percentage
    %   ROH - Remaining Operating Hours
    %   batteryLifeCycle - Estimated remaining battery life cycles
    %   insulationResistance - Insulation resistance in ohms (example constant)
    %   residualCurrentMonitoring - Boolean indicating overcurrent condition
    %   temperatureMonitoring - Monitored temperature value
    %   chargingTime - Estimated charging time in hours

    % Constants for calculations (these values are examples and may need to be adjusted)
    nominalVoltage = 12;        % Nominal voltage of the battery in volts
    maxCurrent = 100;           % Maximum current rating in amperes
    fullChargeCapacity = 100;   % Full charge capacity in Ah
    minVoltageCutoff = 10.5;    % Minimum voltage cutoff for the battery in volts
    maxCycles = 500;            % Estimated maximum cycles for the battery life

    %% 1. Voltage Levels
    voltageLevel = voltage;

    %% 2. Current Levels
    currentLevel = current;

    %% 3. State of Charge (SOC) Calculation
    SOC = (voltage - minVoltageCutoff) / (nominalVoltage - minVoltageCutoff) * 100;
    SOC = max(0, min(SOC, 76));  % Ensure SOC is between 0% and 100%

    %% 4. State of Health (SOH) Calculation (example based on voltage drop)
    SOH = (voltage / nominalVoltage) * 100;

    %% 5. Depth of Discharge (DOD) Calculation
    DOD = 100 - SOC;  % DOD is the complement of SOC

    %% 6. Remaining Operating Hours (ROH) Calculation
    ROH = (fullChargeCapacity - (current / fullChargeCapacity)) * fullChargeCapacity / current; 
    ROH = max(0, ROH);  % Ensure ROH is not negative

    %% 7. Battery Life Cycle Calculation
    batteryLifeCycle = maxCycles * (SOC / 100);  % Estimate remaining cycles based on SOC

    %% 8. Insulation Resistance Calculation (example constant)
    insulationResistance = 1000;  % Example value in ohms

    %% 9. Residual Current Monitoring Calculation (example condition)
    residualCurrentMonitoring = current > maxCurrent;  % True if overcurrent condition

    %% 10. Temperature Monitoring
    temperatureMonitoring = temperature;  % Directly use temperature input

    %% 11. Charging Time Calculation (example)
    chargingTime = (fullChargeCapacity - DOD * fullChargeCapacity / 100) / current; 
end

== matlab function aa_IOT/Subsystem1/MATLAB Function ==
  data: voltage input; voltageLevel output; current input; temperature input; currentLevel output; SOC output; SOH output; DOD output; ROH output; batteryLifeCycle output; insulationResistance output; residualCurrentMonitoring output; temperatureMonitoring output; chargingTime output
function [voltageLevel, currentLevel, SOC, SOH, DOD, ROH, batteryLifeCycle, insulationResistance, residualCurrentMonitoring, temperatureMonitoring, chargingTime] = BatteryParameterEstimation(voltage, current, temperature)
    % BatteryParameterEstimation calculates various battery parameters based on voltage, current, and temperature.
    %
    % Inputs:
    %   voltage - The voltage of the battery in volts
    %   current - The current flowing into the battery in amperes
    %   temperature - The temperature of the battery in degrees Celsius
    %
    % Outputs:
    %   voltageLevel - Monitored voltage level
    %   currentLevel - Monitored current level
    %   SOC - State of Charge as a percentage
    %   SOH - State of Health as a percentage
    %   DOD - Depth of Discharge as a percentage
    %   ROH - Remaining Operating Hours
    %   batteryLifeCycle - Estimated remaining battery life cycles
    %   insulationResistance - Insulation resistance in ohms (example constant)
    %   residualCurrentMonitoring - Boolean indicating overcurrent condition
    %   temperatureMonitoring - Monitored temperature value
    %   chargingTime - Estimated charging time in hours

    % Constants for calculations (these values are examples and may need to be adjusted)
    nominalVoltage = 12;        % Nominal voltage of the battery in volts
    maxCurrent = 100;           % Maximum current rating in amperes
    fullChargeCapacity = 100;   % Full charge capacity in Ah
    minVoltageCutoff = 10.5;    % Minimum voltage cutoff for the battery in volts
    maxCycles = 500;            % Estimated maximum cycles for the battery life

    %% 1. Voltage Levels
    voltageLevel = voltage;

    %% 2. Current Levels
    currentLevel = current;

    %% 3. State of Charge (SOC) Calculation
    SOC = (voltage - minVoltageCutoff) / (nominalVoltage - minVoltageCutoff) * 100;
    SOC = max(0, min(SOC, 100));  % Ensure SOC is between 0% and 100%

    %% 4. State of Health (SOH) Calculation (example based on voltage drop)
    SOH = (voltage / nominalVoltage) * 100;

    %% 5. Depth of Discharge (DOD) Calculation
    DOD = 100 - SOC;  % DOD is the complement of SOC

    %% 6. Remaining Operating Hours (ROH) Calculation
    ROH = (fullChargeCapacity - (current / fullChargeCapacity)) * fullChargeCapacity / current; 
    ROH = max(0, ROH);  % Ensure ROH is not negative

    %% 7. Battery Life Cycle Calculation
    batteryLifeCycle = maxCycles * (SOC / 100);  % Estimate remaining cycles based on SOC

    %% 8. Insulation Resistance Calculation (example constant)
    insulationResistance = 1000;  % Example value in ohms

    %% 9. Residual Current Monitoring Calculation (example condition)
    residualCurrentMonitoring = current > maxCurrent;  % True if overcurrent condition

    %% 10. Temperature Monitoring
    temperatureMonitoring = temperature;  % Directly use temperature input

    %% 11. Charging Time Calculation (example)
    chargingTime = (fullChargeCapacity - DOD * fullChargeCapacity / 100) / current; 
end
